simulink model "FORMATION_CONTROL_trajectory"  (R2024a)
settings: Solver=VariableStepAuto  StartTime=0.0  StopTime=100  RelTol=1e-3
undefined symbols (not defined in the file or in its folder): control_attituded_FO, control_attituded_FO2, control_attituded_FO3, control_position_FO, control_position_FO2, control_position_FO3, Decoupling, Dynamic_UAV, Dynamic_UAV1, Dynamic_UAV2
settings Model: Creator=user  LastModifiedBy=PC05
settings DebuggingCC: UnconnectedInputMsg=warning  UnconnectedOutputMsg=warning  UnconnectedLineMsg=warning
settings ModelReferenceCC: EnableRefExpFcnMdlSchedulingChecks=on
settings RTWCC: GPUComputeCapability=3.5  DLArmComputeVersion=19.05

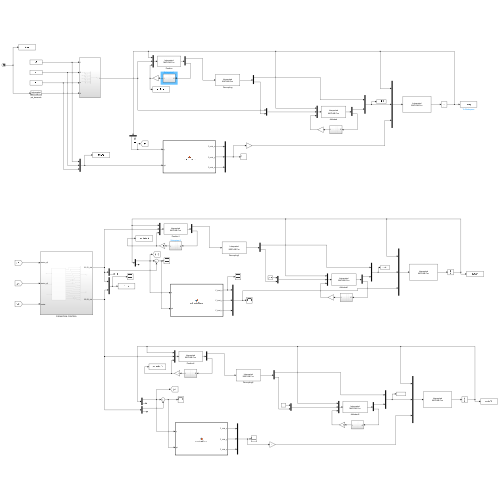
[thumbnail: Simulink's stored preview of the top-level diagram]
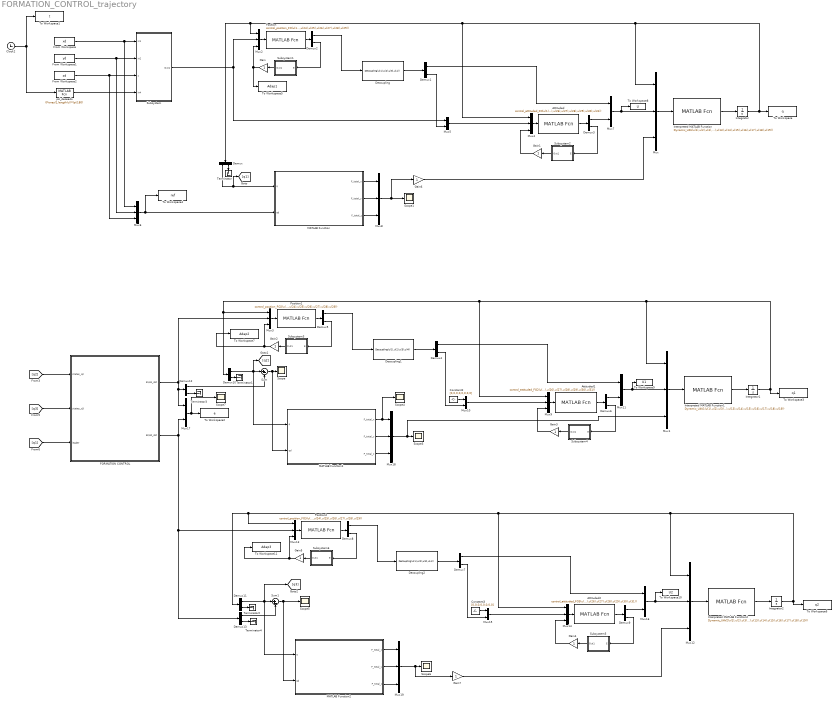
== system FORMATION_CONTROL_trajectory ==
  Attituded : MATLABFcn  MATLABFcn=control_attituded_FO(u(1),u(2),u(3),u(4),u(5),u(6),u(7),u(8),u(9),u(10),u(11),u(12),u(13),u(14),u(15),u(16),u(17),u(18),u(19),u(20),u(21),u(22),u(23),u(24),u(25),u(26),u(27),u(28),u(29),u(30),u(31))  OutputDimensions=9
  Attituded1 : MATLABFcn  MATLABFcn=control_attituded_FO2(u(1),u(2),u(3),u(4),u(5),u(6),u(7),u(8),u(9),u(10),u(11),u(12),u(13),u(14),u(15),u(16),u(17),u(18),u(19),u(20),u(21),u(22),u(23),u(24),u(25),u(26),u(27),u(28),u(29),u(30),u(31))  OutputDimensions=9
  Attituded2 : MATLABFcn  MATLABFcn=control_attituded_FO3(u(1),u(2),u(3),u(4),u(5),u(6),u(7),u(8),u(9),u(10),u(11),u(12),u(13),u(14),u(15),u(16),u(17),u(18),u(19),u(20),u(21),u(22),u(23),u(24),u(25),u(26),u(27),u(28),u(29),u(30),u(31))  OutputDimensions=9
  Clock2 : Clock
  Constant2 : Constant  Value=[0,0,0,0,0,0,0,0]
  Constant3 : Constant  Value=[0,0,0,0,0,0,0,0]
  Decoupling : MATLABFcn  MATLABFcn=Decoupling(u(1),u(2),u(3),u(4))  OutputDimensions=3
  Decoupling1 : MATLABFcn  MATLABFcn=Decoupling(u(1),u(2),u(3),u(4))  OutputDimensions=3
  Decoupling2 : MATLABFcn  MATLABFcn=Decoupling(u(1),u(2),u(3),u(4))  OutputDimensions=3
  Demux : Demux  Outputs=[6 6]
  Demux1 : Demux  Outputs=[1 2]
  Demux10 : Demux  Outputs=[6 6]
  Demux11 : Demux  Outputs=[6 6]
  Demux12 : Demux  Outputs=[6 2]
  Demux13 : Demux  Outputs=[6 2]
  Demux2 : Demux  Outputs=[4 6]
  Demux3 : Demux  Outputs=[3 6]
  Demux4 : Demux  Outputs=[1 2]
  Demux5 : Demux  Outputs=[4 6]
  Demux6 : Demux  Outputs=[3 6]
  Demux7 : Demux  Outputs=[1 2]
  Demux8 : Demux  Outputs=[4 6]
  Demux9 : Demux  Outputs=[3 6]
  FORMATION CONTROL : Subsystem
  From Workspace : FromWorkspace  VariableName=xd  OutDataTypeStr=double
  From Workspace1 : FromWorkspace  VariableName=yd  OutDataTypeStr=double
  From Workspace2 : FromWorkspace  VariableName=zd  OutDataTypeStr=double
  Gain{,1..7} (8 alike) : Gain
  Integrator : Integrator  InitialCondition=[0.5 0.5 0.01 0.01 0.01 0.01 0.01 0.01 0.05 0.01 0.01 0.01]
  Integrator1 : Integrator  InitialCondition=[-1 -2 0.01 0.01 0.01 0.01 0.01 0.01 0.05 0.01 0.01 0.01]
  Integrator2 : Integrator  InitialCondition=[-1 2 0.01 0.01 0.01 0.01 0.01 0.01 0.05 0.01 0.01 0.01]
  Interpreted MATLAB Function : MATLABFcn  MATLABFcn=Dynamic_UAV(u(1),u(2),u(3),u(4),u(5),u(6),u(7),u(8),u(9),u(10),u(11),u(12),u(13),u(14),u(15),u(16),u(17),u(18),u(19))  OutputDimensions=12
  Interpreted MATLAB Function1 : MATLABFcn  MATLABFcn=Dynamic_UAV1(u(1),u(2),u(3),u(4),u(5),u(6),u(7),u(8),u(9),u(10),u(11),u(12),u(13),u(14),u(15),u(16),u(17),u(18),u(19))  OutputDimensions=12
  Interpreted MATLAB Function2 : MATLABFcn  MATLABFcn=Dynamic_UAV2(u(1),u(2),u(3),u(4),u(5),u(6),u(7),u(8),u(9),u(10),u(11),u(12),u(13),u(14),u(15),u(16),u(17),u(18),u(19))  OutputDimensions=12
  MATLAB Function : MATLAB Function  TreatAsAtomicUnit=on
  MATLAB Function1 : MATLAB Function  TreatAsAtomicUnit=on
  MATLAB Function2 : MATLAB Function  TreatAsAtomicUnit=on
  Mux : Mux  Inputs=[12 4 3]
  Mux1 : Mux  Inputs=[12 4 3]
  Mux10 : Mux  Inputs=[8 2]
  Mux11 : Mux  Inputs=[1 3]
  Mux12 : Mux  Inputs=[12 4 3]
  Mux13 : Mux  Inputs=[12 8 9]
  Mux14 : Mux  Inputs=[12 10 9]
  Mux15 : Mux  Inputs=[8 2]
  Mux16 : Mux  Inputs=[1 3]
  Mux17 : Mux  Inputs=2
  Mux{6,8,18..19} (4 alike) : Mux  Inputs=3
  Mux2 : Mux  Inputs=[12 8 9]
  Mux3 : Mux  Inputs=[12 8 9]
  Mux4 : Mux  Inputs=[12 10 9]
  Mux5 : Mux  Inputs=[8 2]
  Mux7 : Mux  Inputs=[1 3]
  Mux9 : Mux  Inputs=[12 10 9]
  Position : MATLABFcn  MATLABFcn=control_position_FO(u(1),u(2),u(3),u(4),u(5),u(6),u(7),u(8),u(9),u(10),u(11),u(12),u(13),u(14),u(15),u(16),u(17),u(18),u(19),u(20),u(21),u(22),u(23),u(24),u(25),u(26),u(27),u(28),u(29))  OutputDimensions=10
  Position1 : MATLABFcn  MATLABFcn=control_position_FO2(u(1),u(2),u(3),u(4),u(5),u(6),u(7),u(8),u(9),u(10),u(11),u(12),u(13),u(14),u(15),u(16),u(17),u(18),u(19),u(20),u(21),u(22),u(23),u(24),u(25),u(26),u(27),u(28),u(29))  OutputDimensions=10
  Position2 : MATLABFcn  MATLABFcn=control_position_FO3(u(1),u(2),u(3),u(4),u(5),u(6),u(7),u(8),u(9),u(10),u(11),u(12),u(13),u(14),u(15),u(16),u(17),u(18),u(19),u(20),u(21),u(22),u(23),u(24),u(25),u(26),u(27),u(28),u(29))  OutputDimensions=10
  Scope{,1,3..7} (7 alike) : Scope
  Subsystem : Subsystem
  Subsystem1 : Subsystem
  Subsystem2 : Subsystem
  Subsystem3 : Subsystem
  Subsystem4 : Subsystem
  Subsystem5 : Subsystem
  Subsystem6 : Subsystem
  Sum : Sum  Inputs=|+-
  Sum1 : Sum  Inputs=|+-
  Terminator{,1..4} (5 alike) : Terminator
  To Workspace : ToWorkspace  VariableName=q  SampleTime=-1
  To Workspace1 : ToWorkspace  VariableName=t  SampleTime=-1
  To Workspace10 : ToWorkspace  VariableName=U2  SampleTime=-1
  To Workspace11 : ToWorkspace  VariableName=Adap3  SampleTime=-1
  To Workspace2 : ToWorkspace  VariableName=e  SampleTime=-1
  To Workspace3 : ToWorkspace  VariableName=q1  SampleTime=-1
  To Workspace4 : ToWorkspace  VariableName=ref  SampleTime=-1
  To Workspace5 : ToWorkspace  VariableName=Adap1  SampleTime=-1
  To Workspace6 : ToWorkspace  VariableName=q2  SampleTime=-1
  To Workspace7 : ToWorkspace  VariableName=Adap2  SampleTime=-1
  To Workspace8 : ToWorkspace  VariableName=U  SampleTime=-1
  To Workspace9 : ToWorkspace  VariableName=U1  SampleTime=-1
  psi_deseado : MATLABFcn  MATLABFcn=0*ones(1,length(u))*(pi/180)
  wires:
  Mux/1 -> Interpreted MATLAB Function/1
  Interpreted MATLAB Function/1 -> Integrator/1
  Integrator/1 -> To Workspace/1, Demux/1, Mux2/1, Mux4/1, Mux/1
  From Workspace/1 -> Subsystem/1(In1), Mux6/1
  From Workspace1/1 -> Mux6/2, Subsystem/2(In2)
  From Workspace2/1 -> Subsystem/3(z), Mux6/3
  psi_deseado/1 -> Subsystem/4(In4)
  Mux2/1 -> Position/1
  Decoupling/1 -> Demux1/1
  Mux5/1 -> Mux4/2
  Demux1/1 -> Mux7/1
  Mux7/1 -> To Workspace8/1, Mux/2
  Demux1/2 -> Mux5/2
  Clock2/1 -> psi_deseado/1, To Workspace1/1
  Demux/2 -> Terminator/1
  Demux/1 -> [q1], MATLAB Function/1(q)
  Mux6/1 -> To Workspace4/1, MATLAB Function/2(qd)
  MATLAB Function/1(F_total_x) -> Mux8/1
  MATLAB Function/2(F_total_y) -> Mux8/2
  MATLAB Function/3(F_total_z) -> Mux8/3
  Demux2/1 -> Decoupling/1
  Position/1 -> Demux2/1
  Mux4/1 -> Attituded/1
  Attituded/1 -> Demux3/1
  Demux3/1 -> Mux7/2
  [q1] -> FORMATION CONTROL/3(leader)
  [q3] -> FORMATION CONTROL/2(states_q3)
  [q2] -> FORMATION CONTROL/1(states_q2)
  Decoupling1/1 -> Demux4/1
  Interpreted MATLAB Function1/1 -> Integrator1/1
  Mux1/1 -> Interpreted MATLAB Function1/1
  Demux4/1 -> Mux11/1
  Mux18/1 -> Mux1/3, Scope3/1
  Demux4/2 -> Mux10/2
  Mux11/1 -> To Workspace9/1, Mux1/2
  Decoupling2/1 -> Demux7/1
  Interpreted MATLAB Function2/1 -> Integrator2/1
  Subsystem/1(Out1) -> Mux5/1, Mux2/2
  Mux12/1 -> Interpreted MATLAB Function2/1
  Demux7/1 -> Mux16/1
  Mux19/1 -> Gain7/1, Scope6/1
  Demux7/2 -> Mux15/2
  Mux16/1 -> Mux12/2, To Workspace10/1
  Demux10/2 -> Terminator1/1
  Demux10/1 -> MATLAB Function1/1(q), [q2], Sum/1
  Demux11/1 -> MATLAB Function2/1(q), [q3], Sum1/1
  Demux11/2 -> Terminator2/1
  Constant2/1 -> Mux10/1
  Constant3/1 -> Mux15/1
  Mux17/1 -> Scope7/1, To Workspace2/1
  Sum/1 -> MATLAB Function1/2(qd), Scope/1
  Demux12/1 -> Sum/2
  Demux12/2 -> Terminator3/1
  MATLAB Function1/2(F_total_y) -> Mux18/2
  MATLAB Function1/1(F_total_x) -> Scope4/1, Mux18/1
  MATLAB Function1/3(F_total_z) -> Mux18/3
  Demux13/2 -> Terminator4/1
  Sum1/1 -> MATLAB Function2/2(qd), Scope5/1
  Demux13/1 -> Sum1/2
  MATLAB Function2/2(F_total_y) -> Mux19/2
  MATLAB Function2/3(F_total_z) -> Mux19/3
  MATLAB Function2/1(F_total_x) -> Mux19/1
  Demux2/2 -> Subsystem1/1(E)
  Subsystem1/1(Out1) -> Gain/1
  Gain/1 -> To Workspace5/1, Mux2/3
  Subsystem2/1(Out1) -> Gain1/1
  Demux3/2 -> Subsystem2/1(E)
  Gain1/1 -> Mux4/3
  Subsystem3/1(Out1) -> Gain2/1
  Gain2/1 -> To Workspace7/1, Mux3/3
  FORMATION CONTROL/1(E1,E1_dot) -> Demux12/1, Mux17/1, Mux3/2
  Position1/1 -> Demux5/1
  Mux3/1 -> Position1/1
  Demux5/2 -> Subsystem3/1(E)
  Demux5/1 -> Decoupling1/1
  Gain3/1 -> Mux9/3
  Demux6/1 -> Mux11/2
  Demux6/2 -> Subsystem4/1(E)
  Mux9/1 -> Attituded1/1
  Attituded1/1 -> Demux6/1
  Subsystem4/1(Out1) -> Gain3/1
  Mux10/1 -> Mux9/2
  Integrator1/1 -> To Workspace3/1, Mux9/1, Mux3/1, Demux10/1, Mux1/1
  Gain4/1 -> Mux14/3
  Demux9/1 -> Mux16/2
  Demux9/2 -> Subsystem5/1(E)
  Mux14/1 -> Attituded2/1
  Attituded2/1 -> Demux9/1
  Subsystem5/1(Out1) -> Gain4/1
  Mux15/1 -> Mux14/2
  FORMATION CONTROL/2(E2,E2_dot) -> Demux13/1, Mux13/2, Mux17/2
  Integrator2/1 -> To Workspace6/1, Mux14/1, Mux13/1, Demux11/1, Mux12/1
  Mux13/1 -> Position2/1
  Demux8/2 -> Subsystem6/1(E)
  Demux8/1 -> Decoupling2/1
  Gain5/1 -> To Workspace11/1, Mux13/3
  Position2/1 -> Demux8/1
  Subsystem6/1(Out1) -> Gain5/1
  Mux8/1 -> Scope1/1, Gain6/1
  Gain6/1 -> Mux/3
  Gain7/1 -> Mux12/3

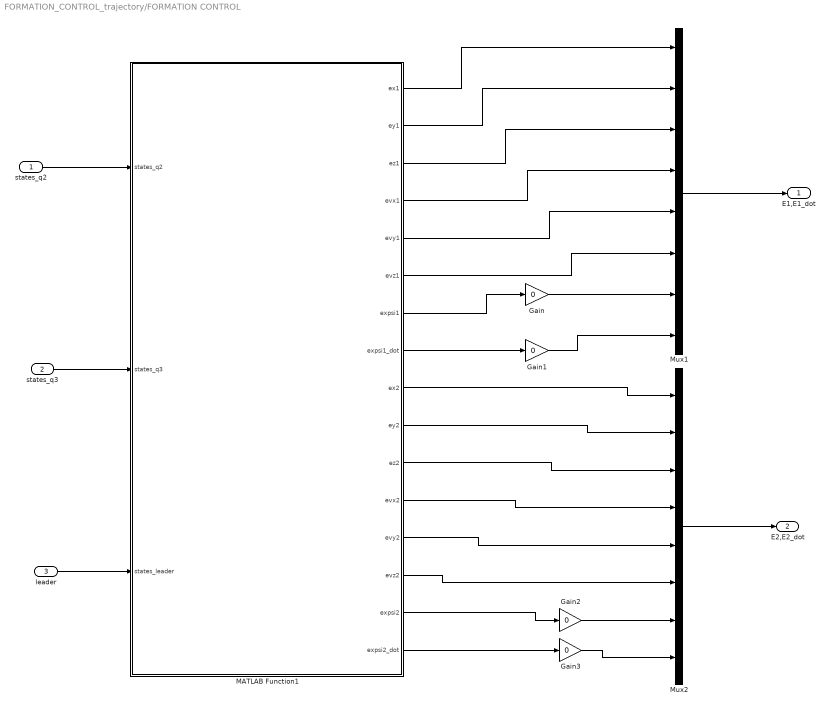
== system FORMATION_CONTROL_trajectory/FORMATION CONTROL ==
  states_q2 : Inport
  states_q3 : Inport  Port=2
  leader : Inport  Port=3
  Gain{,1..3} (4 alike) : Gain  Gain=0
  MATLAB Function1 : MATLAB Function  TreatAsAtomicUnit=on
  Mux1 : Mux  Inputs=8
  Mux2 : Mux  Inputs=8
  E1,E1_dot : Outport
  E2,E2_dot : Outport  Port=2
  wires:
  Mux1/1 -> E1,E1_dot/1
  states_q2/1 -> MATLAB Function1/1(states_q2)
  states_q3/1 -> MATLAB Function1/2(states_q3)
  leader/1 -> MATLAB Function1/3(states_leader)
  MATLAB Function1/1(ex1) -> Mux1/1
  MATLAB Function1/2(ey1) -> Mux1/2
  MATLAB Function1/3(ez1) -> Mux1/3
  MATLAB Function1/4(evx1) -> Mux1/4
  MATLAB Function1/5(evy1) -> Mux1/5
  MATLAB Function1/6(evz1) -> Mux1/6
  MATLAB Function1/14(evz2) -> Mux2/6
  MATLAB Function1/11(ez2) -> Mux2/3
  MATLAB Function1/9(ex2) -> Mux2/1
  MATLAB Function1/12(evx2) -> Mux2/4
  Mux2/1 -> E2,E2_dot/1
  MATLAB Function1/10(ey2) -> Mux2/2
  MATLAB Function1/13(evy2) -> Mux2/5
  MATLAB Function1/7(expsi1) -> Gain/1
  MATLAB Function1/8(expsi1_dot) -> Gain1/1
  MATLAB Function1/15(expsi2) -> Gain2/1
  MATLAB Function1/16(expsi2_dot) -> Gain3/1
  Gain/1 -> Mux1/7
  Gain1/1 -> Mux1/8
  Gain2/1 -> Mux2/7
  Gain3/1 -> Mux2/8

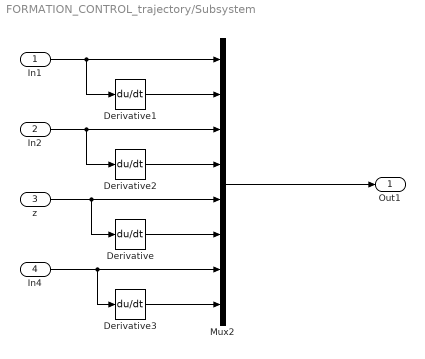
== system FORMATION_CONTROL_trajectory/Subsystem ==
  In1 : Inport
  In2 : Inport  Port=2
  z : Inport  Port=3
  In4 : Inport  Port=4
  Derivative{,1..3} (4 alike) : Derivative
  Mux2 : Mux  Inputs=8
  Out1 : Outport
  wires:
  In2/1 -> Mux2/3, Derivative2/1
  Derivative/1 -> Mux2/6
  z/1 -> Mux2/5, Derivative/1
  Derivative3/1 -> Mux2/8
  In4/1 -> Mux2/7, Derivative3/1
  In1/1 -> Mux2/1, Derivative1/1
  Derivative2/1 -> Mux2/4
  Derivative1/1 -> Mux2/2
  Mux2/1 -> Out1/1

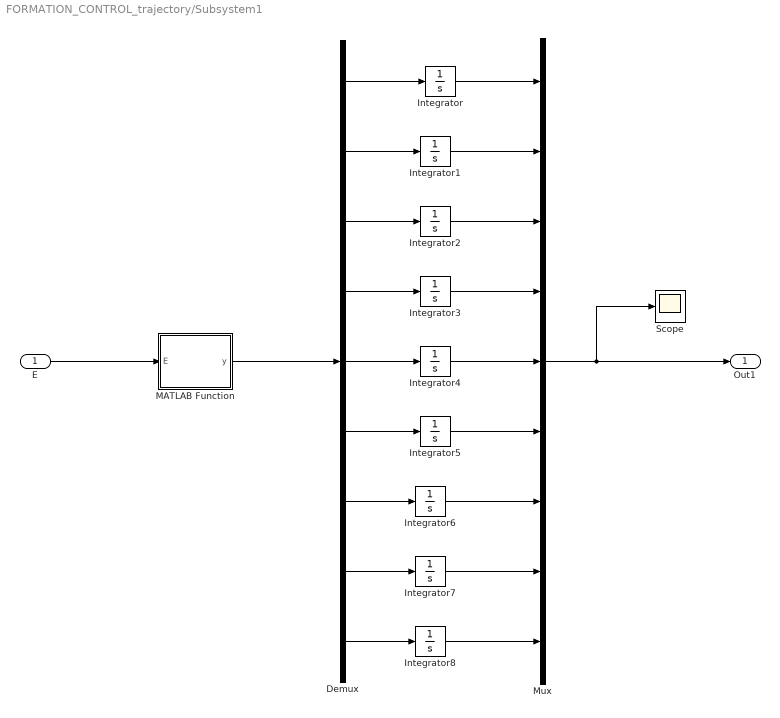
== system FORMATION_CONTROL_trajectory/Subsystem1 ==
  E : Inport
  Demux : Demux  Outputs=9
  Integrator{,1..8} (9 alike) : Integrator  InitialCondition=0.01
  MATLAB Function : MATLAB Function  TreatAsAtomicUnit=on
  Mux : Mux  Inputs=9
  Scope : Scope
  Out1 : Outport
  wires:
  Mux/1 -> Scope/1, Out1/1
  E/1 -> MATLAB Function/1(E)
  MATLAB Function/1(y) -> Demux/1
  Integrator/1 -> Mux/1
  Demux/1 -> Integrator/1
  Demux/2 -> Integrator1/1
  Integrator1/1 -> Mux/2
  Demux/3 -> Integrator2/1
  Integrator2/1 -> Mux/3
  Demux/4 -> Integrator3/1
  Integrator3/1 -> Mux/4
  Demux/5 -> Integrator4/1
  Integrator4/1 -> Mux/5
  Demux/6 -> Integrator5/1
  Integrator5/1 -> Mux/6
  Demux/7 -> Integrator6/1
  Integrator6/1 -> Mux/7
  Demux/8 -> Integrator7/1
  Integrator7/1 -> Mux/8
  Demux/9 -> Integrator8/1
  Integrator8/1 -> Mux/9

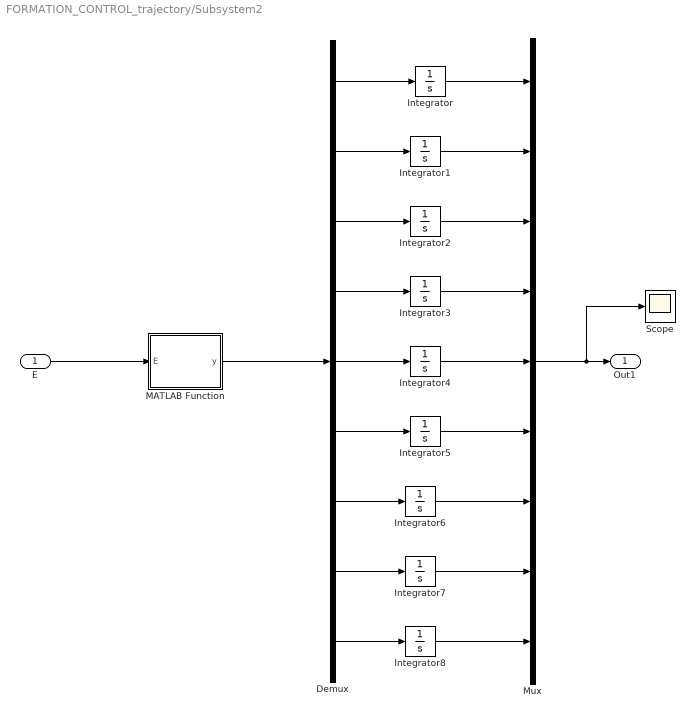
== system FORMATION_CONTROL_trajectory/Subsystem2 ==
  E : Inport
  Demux : Demux  Outputs=9
  Integrator{,1..8} (9 alike) : Integrator  InitialCondition=0.01
  MATLAB Function : MATLAB Function  TreatAsAtomicUnit=on
  Mux : Mux  Inputs=9
  Scope : Scope
  Out1 : Outport
  wires:
  Demux/5 -> Integrator4/1
  Integrator3/1 -> Mux/4
  Integrator6/1 -> Mux/7
  Demux/8 -> Integrator7/1
  Integrator5/1 -> Mux/6
  Integrator4/1 -> Mux/5
  Demux/9 -> Integrator8/1
  Demux/6 -> Integrator5/1
  Integrator8/1 -> Mux/9
  Integrator7/1 -> Mux/8
  Demux/7 -> Integrator6/1
  Demux/4 -> Integrator3/1
  Integrator2/1 -> Mux/3
  Demux/3 -> Integrator2/1
  Demux/1 -> Integrator/1
  Mux/1 -> Scope/1, Out1/1
  Integrator/1 -> Mux/1
  Integrator1/1 -> Mux/2
  Demux/2 -> Integrator1/1
  E/1 -> MATLAB Function/1(E)
  MATLAB Function/1(y) -> Demux/1

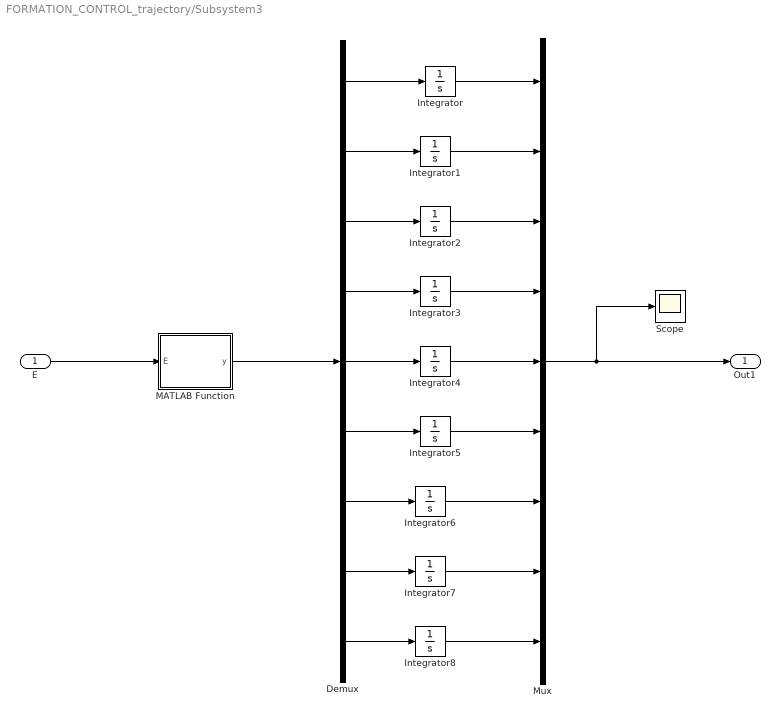
== system FORMATION_CONTROL_trajectory/Subsystem3 ==
  E : Inport
  Demux : Demux  Outputs=9
  Integrator{,1..8} (9 alike) : Integrator  InitialCondition=0.01
  MATLAB Function : MATLAB Function  TreatAsAtomicUnit=on
  Mux : Mux  Inputs=9
  Scope : Scope
  Out1 : Outport
  wires:
  Mux/1 -> Scope/1, Out1/1
  E/1 -> MATLAB Function/1(E)
  MATLAB Function/1(y) -> Demux/1
  Integrator/1 -> Mux/1
  Demux/1 -> Integrator/1
  Demux/2 -> Integrator1/1
  Integrator1/1 -> Mux/2
  Demux/3 -> Integrator2/1
  Integrator2/1 -> Mux/3
  Demux/4 -> Integrator3/1
  Integrator3/1 -> Mux/4
  Demux/5 -> Integrator4/1
  Integrator4/1 -> Mux/5
  Demux/6 -> Integrator5/1
  Integrator5/1 -> Mux/6
  Demux/7 -> Integrator6/1
  Integrator6/1 -> Mux/7
  Demux/8 -> Integrator7/1
  Integrator7/1 -> Mux/8
  Demux/9 -> Integrator8/1
  Integrator8/1 -> Mux/9

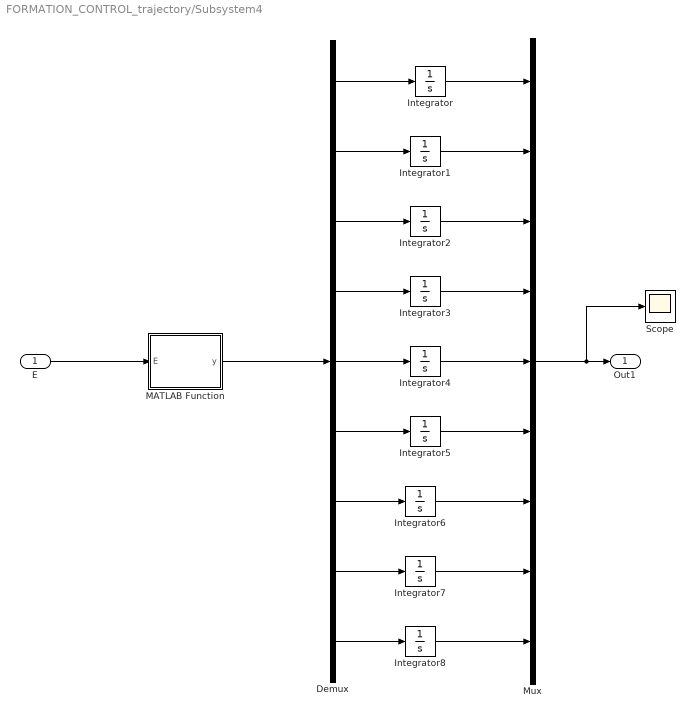
== system FORMATION_CONTROL_trajectory/Subsystem4 ==
  E : Inport
  Demux : Demux  Outputs=9
  Integrator{,1..8} (9 alike) : Integrator  InitialCondition=0.01
  MATLAB Function : MATLAB Function  TreatAsAtomicUnit=on
  Mux : Mux  Inputs=9
  Scope : Scope
  Out1 : Outport
  wires:
  Demux/5 -> Integrator4/1
  Integrator3/1 -> Mux/4
  Integrator6/1 -> Mux/7
  Demux/8 -> Integrator7/1
  Integrator5/1 -> Mux/6
  Integrator4/1 -> Mux/5
  Demux/9 -> Integrator8/1
  Demux/6 -> Integrator5/1
  Integrator8/1 -> Mux/9
  Integrator7/1 -> Mux/8
  Demux/7 -> Integrator6/1
  Demux/4 -> Integrator3/1
  Integrator2/1 -> Mux/3
  Demux/3 -> Integrator2/1
  Demux/1 -> Integrator/1
  Mux/1 -> Scope/1, Out1/1
  Integrator/1 -> Mux/1
  Integrator1/1 -> Mux/2
  Demux/2 -> Integrator1/1
  E/1 -> MATLAB Function/1(E)
  MATLAB Function/1(y) -> Demux/1

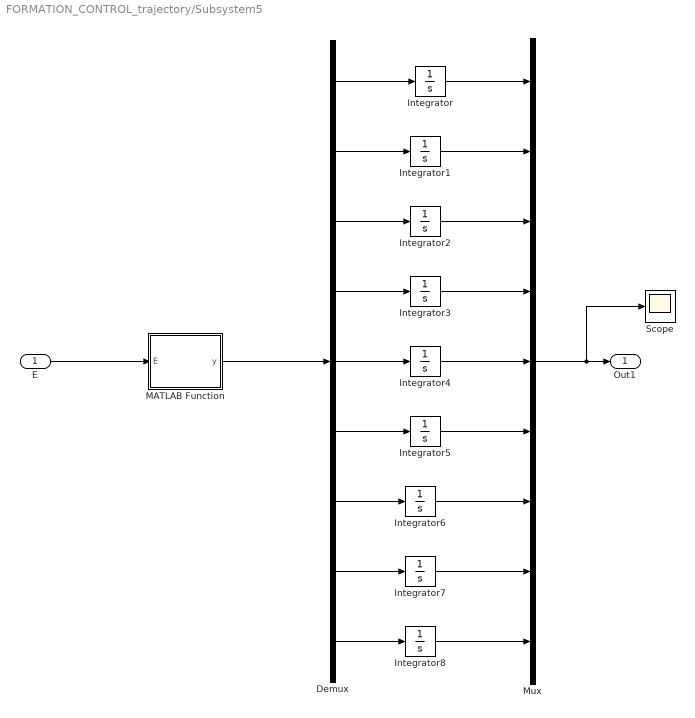
== system FORMATION_CONTROL_trajectory/Subsystem5 ==
  E : Inport
  Demux : Demux  Outputs=9
  Integrator{,1..8} (9 alike) : Integrator  InitialCondition=0.01
  MATLAB Function : MATLAB Function  TreatAsAtomicUnit=on
  Mux : Mux  Inputs=9
  Scope : Scope
  Out1 : Outport
  wires:
  Demux/5 -> Integrator4/1
  Integrator3/1 -> Mux/4
  Integrator6/1 -> Mux/7
  Demux/8 -> Integrator7/1
  Integrator5/1 -> Mux/6
  Integrator4/1 -> Mux/5
  Demux/9 -> Integrator8/1
  Demux/6 -> Integrator5/1
  Integrator8/1 -> Mux/9
  Integrator7/1 -> Mux/8
  Demux/7 -> Integrator6/1
  Demux/4 -> Integrator3/1
  Integrator2/1 -> Mux/3
  Demux/3 -> Integrator2/1
  Demux/1 -> Integrator/1
  Mux/1 -> Scope/1, Out1/1
  Integrator/1 -> Mux/1
  Integrator1/1 -> Mux/2
  Demux/2 -> Integrator1/1
  E/1 -> MATLAB Function/1(E)
  MATLAB Function/1(y) -> Demux/1

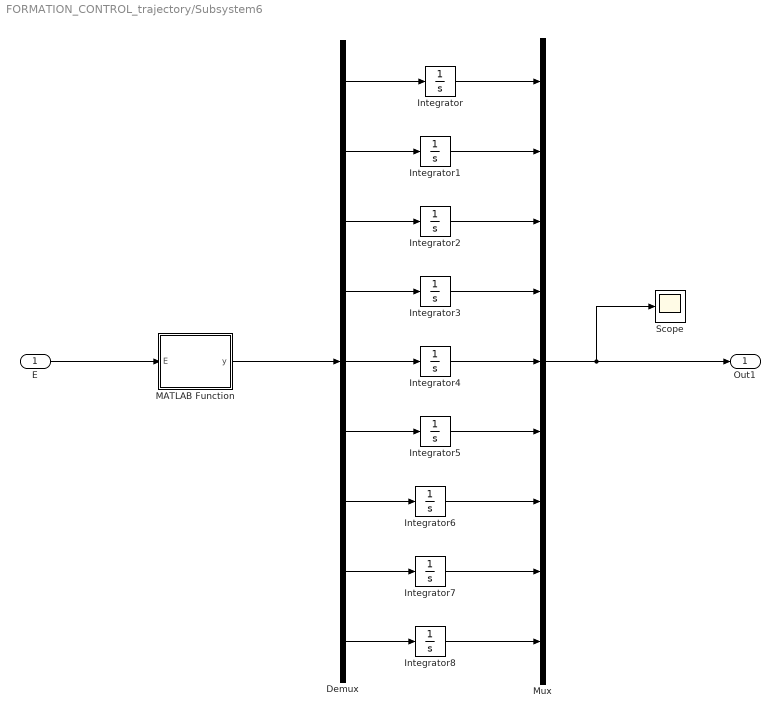
== system FORMATION_CONTROL_trajectory/Subsystem6 ==
  E : Inport
  Demux : Demux  Outputs=9
  Integrator{,1..8} (9 alike) : Integrator  InitialCondition=0.01
  MATLAB Function : MATLAB Function  TreatAsAtomicUnit=on
  Mux : Mux  Inputs=9
  Scope : Scope
  Out1 : Outport
  wires:
  Mux/1 -> Scope/1, Out1/1
  E/1 -> MATLAB Function/1(E)
  MATLAB Function/1(y) -> Demux/1
  Integrator/1 -> Mux/1
  Demux/1 -> Integrator/1
  Demux/2 -> Integrator1/1
  Integrator1/1 -> Mux/2
  Demux/3 -> Integrator2/1
  Integrator2/1 -> Mux/3
  Demux/4 -> Integrator3/1
  Integrator3/1 -> Mux/4
  Demux/5 -> Integrator4/1
  Integrator4/1 -> Mux/5
  Demux/6 -> Integrator5/1
  Integrator5/1 -> Mux/6
  Demux/7 -> Integrator6/1
  Integrator6/1 -> Mux/7
  Demux/8 -> Integrator7/1
  Integrator7/1 -> Mux/8
  Demux/9 -> Integrator8/1
  Integrator8/1 -> Mux/9

== matlab function FORMATION_CONTROL_trajectory/MATLAB Function2 ==
  data: q input; F_total_x output; qd input; F_total_y output; F_total_z output
function [F_total_x, F_total_y, F_total_z] = calculateFtotal(q, qd)
    % q: Posición actual del cuadricóptero [x, y, z]
    % qd: Posición de referencia [xd, yd, zd]
    % obs: Posición de los obstáculos [xo, yo, zo]
    % k_att: Constante de proporcionalidad para la fuerza atractiva
    % k_rep: Constante de proporcionalidad para la fuerza repulsiva
    % rho_0: Umbral de influencia del obstáculo
    
    k_att = 3; % constante del campo atractivo
    k_repx = 0.5; % constante del campo repulsivo
    k_repy = 0.5; % constante del campo repulsivo
    k_repz = 0; % constante del campo repulsivo
    rho_0 = 1; % radio de influencia del obstáculo

    % Definición de obstáculos (tres obstáculos)
    obstacles = [
       5.8, 3.5, 4;  % Obstacle 1
        0, 0, 0;  % Obstacle 2
        6, 13, 4   % Obstacle 3
    ];

    x = q(1);
    y = q(2);
    z = q(3);
    xd = qd(1);
    yd = qd(2);
    zd = qd(3);

    % Calcular la fuerza atractiva
    F_attX = -k_att * (x - xd);
    F_attY = -k_att * (y - yd);
    F_attZ = -k_att * (z - zd);

    % Inicializar la fuerza repulsiva a cero
    F_repX = 0;
    F_repY = 0;
    F_repZ = 0;

    % Calcular la fuerza repulsiva para cada obstáculo
    for i = 1:size(obstacles, 1)
        obs = obstacles(i, :);
        rho = sqrt((x - obs(1))^2 + (y - obs(2))^2 + (z - obs(3))^2);
        
        if rho <= rho_0
            directionX = (x - obs(1)) / rho;
            directionY = (y - obs(2)) / rho;
            directionZ = (z - obs(3)) / rho;
            F_repX = F_repX + k_repx * (1/rho - 1/rho_0) * (1/rho^2) * directionX;
            F_repY = F_repY + k_repy * (1/rho - 1/rho_0) * (1/rho^2) * directionY;
            F_repZ = F_repZ + k_repz * (1/rho - 1/rho_0) * (1/rho^2) * directionZ;
        end
    end

    F_total_x = (F_attX + F_repX);
    F_total_y = (F_attY + F_repY);
    F_total_z = (F_attZ + F_repZ);
    
end

== matlab function FORMATION_CONTROL_trajectory/FORMATION CONTROL/MATLAB Function1 ==
  data: states_q2 input; states_q3 input; states_leader input; ex1 output; ey1 output; ez1 output; evx1 output; evy1 output; evz1 output; expsi1 output; expsi1_dot output; ex2 output; ey2 output; ez2 output; evx2 output; evy2 output; evz2 output; expsi2 output; expsi2_dot output
function [ex1,ey1,ez1,evx1,evy1,evz1,expsi1,expsi1_dot,ex2,ey2,ez2,evx2,evy2,evz2,expsi2,expsi2_dot] = formation_control(states_q2,states_q3,states_leader)
x2=states_q2(1);
y2=states_q2(2);
z2=states_q2(3);
Vx2=states_q2(4);
Vy2=states_q2(5);
Vz2=states_q2(6);
x3=states_q3(1);
y3=states_q3(2);
z3=states_q3(3);
Vx3=states_q3(4);
Vy3=states_q3(5);
Vz3=states_q3(6);
x0=states_leader(1);
y0=states_leader(2);
z0=states_leader(3);
Vx0=states_leader(4);
Vy0=states_leader(5);
Vz0=states_leader(6);


p=[x2,y2,z2,x3,y3,z3]';
v=[Vx2,Vy2,Vz2,Vx3,Vy3,Vz3]';
p0=[x0 y0 z0]';
v0=[Vx0 Vy0 Vz0]';
h1=[0, -1, 0];
h2=[ 0, 1, 0];
h=[h1,h2]';
L=[0 0;-1 1];
B=[1 0; 0 0];
LB=L+B;
p_=p - kron(ones(2,1),p0) - h;
ep_=p_;

v_= v - kron(ones(2,1),v0);
ev_=v_;

ex1=ep_(1);
ey1=ep_(2);
ez1=ep_(3);
evx1=ev_(1);
evy1=ev_(2);
evz1=ev_(3);
expsi1=ex1*0;
expsi1_dot=ex1*0;


ex2=ep_(4);
ey2=ep_(5);
ez2=ep_(6);
evx2=ev_(4);
evy2=ev_(5);
evz2=ev_(6);
expsi2=ex2*0;
expsi2_dot=ex2*0;
end

== matlab function FORMATION_CONTROL_trajectory/MATLAB Function1 ==
  data: q input; F_total_x output; qd input; F_total_y output; F_total_z output
function [F_total_x, F_total_y, F_total_z] = calculateFtotal(q, qd)
    % q: Posición actual del cuadricóptero [x, y, z]
    % qd: Posición de referencia [xd, yd, zd]
    % obs: Posición de los obstáculos [xo, yo, zo]
    % k_att: Constante de proporcionalidad para la fuerza atractiva
    % k_rep: Constante de proporcionalidad para la fuerza repulsiva
    % rho_0: Umbral de influencia del obstáculo
    
    k_att = 3; % constante del campo atractivo
    k_repx = 0.5; % constante del campo repulsivo
    k_repy = 0.5; % constante del campo repulsivo
    k_repz = 0; % constante del campo repulsivo
    rho_0 = 1; % radio de influencia del obstáculo

    % Definición de obstáculos (tres obstáculos)
    obstacles = [
        0, 0, 0;  % Obstacle 1
        6, 8, 4;  % Obstacle 2
        0, 0, 0   % Obstacle 3
    ];

    x = q(1);
    y = q(2);
    z = q(3);
    xd = qd(1);
    yd = qd(2);
    zd = qd(3);

    % Calcular la fuerza atractiva
    F_attX = -k_att * (x - xd);
    F_attY = -k_att * (y - yd);
    F_attZ = -k_att * (z - zd);

    % Inicializar la fuerza repulsiva a cero
    F_repX = 0;
    F_repY = 0;
    F_repZ = 0;

    % Calcular la fuerza repulsiva para cada obstáculo
    for i = 1:size(obstacles, 1)
        obs = obstacles(i, :);
        rho = sqrt((x - obs(1))^2 + (y - obs(2))^2 + (z - obs(3))^2);
        
        if rho <= rho_0
            directionX = (x - obs(1)) / rho;
            directionY = (y - obs(2)) / rho;
            directionZ = (z - obs(3)) / rho;
            F_repX = F_repX + k_repx * (1/rho - 1/rho_0) * (1/rho^2) * directionX;
            F_repY = F_repY + k_repy * (1/rho - 1/rho_0) * (1/rho^2) * directionY;
            F_repZ = F_repZ + k_repz * (1/rho - 1/rho_0) * (1/rho^2) * directionZ;
        end
    end

    F_total_x = (F_attX + F_repX);
    F_total_y = (F_attY + F_repY);
    F_total_z = (F_attZ + F_repZ);
    
end

== matlab function FORMATION_CONTROL_trajectory/MATLAB Function ==
  data: q input; F_total_x output; qd input; F_total_y output; F_total_z output
function [F_total_x, F_total_y, F_total_z] = calculateFtotal(q, qd)
    % q: Posición actual del cuadricóptero [x, y, z]
    % qd: Posición de referencia [xd, yd, zd]
    % obs: Posición de los obstáculos [xo, yo, zo]
    % k_att: Constante de proporcionalidad para la fuerza atractiva
    % k_rep: Constante de proporcionalidad para la fuerza repulsiva
    % rho_0: Umbral de influencia del obstáculo
    
    k_att = 3; % constante del campo atractivo
    k_repx = 0.05; % constante del campo repulsivo
    k_repy = 0.05; % constante del campo repulsivo
    k_repz = 0; % constante del campo repulsivo
    rho_0 = 1; % radio de influencia del obstáculo

    % Definición de obstáculos (tres obstáculos)
    obstacles = [
        6, 3, 4;  % Obstacle 1
        0, 0, 0;  % Obstacle 2
        0, 0, 0   % Obstacle 3
    ];

    x = q(1);
    y = q(2);
    z = q(3);
    xd = qd(1);
    yd = qd(2);
    zd = qd(3);

    % Calcular la fuerza atractiva
    F_attX = -k_att * (x - xd);
    F_attY = -k_att * (y - yd);
    F_attZ = -k_att * (z - zd);

    % Inicializar la fuerza repulsiva a cero
    F_repX = 0;
    F_repY = 0;
    F_repZ = 0;

    % Calcular la fuerza repulsiva para cada obstáculo
    for i = 1:size(obstacles, 1)
        obs = obstacles(i, :);
        rho = sqrt((x - obs(1))^2 + (y - obs(2))^2 + (z - obs(3))^2);
        
        if rho <= rho_0
            directionX = (x - obs(1)) / rho;
            directionY = (y - obs(2)) / rho;
            directionZ = (z - obs(3)) / rho;
            F_repX = F_repX + k_repx * (1/rho - 1/rho_0) * (1/rho^2) * directionX;
            F_repY = F_repY + k_repy * (1/rho - 1/rho_0) * (1/rho^2) * directionY;
            F_repZ = F_repZ + k_repz * (1/rho - 1/rho_0) * (1/rho^2) * directionZ;
        end
    end

    F_total_x = (F_attX + F_repX);
    F_total_y = (F_attY + F_repY);
    F_total_z = (F_attZ + F_repZ);
    
end

== matlab function FORMATION_CONTROL_trajectory/Subsystem1/MATLAB Function ==
  data: E input; y output
function y = FOSMC(E)

ex=E(1);
ey=E(2);
ez=E(3);
sx=E(4);
sy=E(5);
sz=E(6);

Ix_fo=(0.05*(abs(ex)^0.3)*tanh(ex));
Iy_fo=(0.05*(abs(ey)^0.3)*tanh(ey));
Iz_fo=(0.05*(abs(ez)^0.3)*tanh(ez));
k1x_est=3*abs(sx)^(2);
k2x_est=3*abs(sx)^(1.2);
k1y_est=3*abs(sy)^(2);
k2y_est=3*abs(sy)^(1.2);
k1z_est=3*abs(sz)^(2);
k2z_est=3*abs(sz)^(1.2);

y = [Ix_fo,Iy_fo,Iz_fo,k1x_est*0.1,k2x_est*0.1,k1y_est*0.1,k2y_est*0.1,k1z_est*0.05,k2z_est*0.05];

== matlab function FORMATION_CONTROL_trajectory/Subsystem2/MATLAB Function ==
  data: E input; y output
function y = FOSMC(E)

ex=E(1);
ey=E(2);
ez=E(3);
sx=E(4);
sy=E(5);
sz=E(6);

Ix_fo=(0.0002*(abs(ex)^1.2)*tanh(ex));
Iy_fo=(0.0002*(abs(ey)^1.2)*tanh(ey));
Iz_fo=(0.0002*(abs(ez)^1.2)*tanh(ez));
k1x_est=2*abs(sx)^(2);
k2x_est=1.67*abs(sx)^(1.2);
k1y_est=2*abs(sy)^(2);
k2y_est=1.67*abs(sy)^(1.2);
k1z_est=2*abs(sz)^(2);
k2z_est=1.67*abs(sz)^(1.2);

y = [Ix_fo,Iy_fo,Iz_fo,1*k1x_est,1*k2x_est,1*k1y_est,1*k2y_est,1*k1z_est,1*k2z_est];

== matlab function FORMATION_CONTROL_trajectory/Subsystem3/MATLAB Function ==
  data: E input; y output
function y = FOSMC(E)

ex=E(1);
ey=E(2);
ez=E(3);
sx=E(4);
sy=E(5);
sz=E(6);

Ix_fo=(0.05*(abs(ex)^0.3)*tanh(ex));
Iy_fo=(0.05*(abs(ey)^0.3)*tanh(ey));
Iz_fo=(0.05*(abs(ez)^0.3)*tanh(ez));
k1x_est=3*abs(sx)^(2);
k2x_est=3*abs(sx)^(1.2);
k1y_est=3*abs(sy)^(2);
k2y_est=3*abs(sy)^(1.2);
k1z_est=3*abs(sz)^(2);
k2z_est=3*abs(sz)^(1.2);

y = [Ix_fo,Iy_fo,Iz_fo,k1x_est*0.1,k2x_est*0.1,k1y_est*0.1,k2y_est*0.1,k1z_est*0.05,k2z_est*0.05];

== matlab function FORMATION_CONTROL_trajectory/Subsystem4/MATLAB Function ==
  data: E input; y output
function y = FOSMC(E)

ex=E(1);
ey=E(2);
ez=E(3);
sx=E(4);
sy=E(5);
sz=E(6);

Ix_fo=(0.0002*(abs(ex)^1.2)*tanh(ex));
Iy_fo=(0.0002*(abs(ey)^1.2)*tanh(ey));
Iz_fo=(0.0002*(abs(ez)^1.2)*tanh(ez));
k1x_est=2*abs(sx)^(2);
k2x_est=1.67*abs(sx)^(1.2);
k1y_est=2*abs(sy)^(2);
k2y_est=1.67*abs(sy)^(1.2);
k1z_est=2*abs(sz)^(2);
k2z_est=1.67*abs(sz)^(1.2);

y = [Ix_fo,Iy_fo,Iz_fo,1*k1x_est,1*k2x_est,1*k1y_est,1*k2y_est,1*k1z_est,1*k2z_est];

== matlab function FORMATION_CONTROL_trajectory/Subsystem5/MATLAB Function ==
  data: E input; y output
function y = FOSMC(E)

ex=E(1);
ey=E(2);
ez=E(3);
sx=E(4);
sy=E(5);
sz=E(6);

Ix_fo=(0.0002*(abs(ex)^1.2)*tanh(ex));
Iy_fo=(0.0002*(abs(ey)^1.2)*tanh(ey));
Iz_fo=(0.0002*(abs(ez)^1.2)*tanh(ez));
k1x_est=2*abs(sx)^(2);
k2x_est=1.67*abs(sx)^(1.2);
k1y_est=2*abs(sy)^(2);
k2y_est=1.67*abs(sy)^(1.2);
k1z_est=2*abs(sz)^(2);
k2z_est=1.67*abs(sz)^(1.2);

y = [Ix_fo,Iy_fo,Iz_fo,1*k1x_est,1*k2x_est,1*k1y_est,1*k2y_est,1*k1z_est,1*k2z_est];

== matlab function FORMATION_CONTROL_trajectory/Subsystem6/MATLAB Function ==
  data: E input; y output
function y = FOSMC(E)

ex=E(1);
ey=E(2);
ez=E(3);
sx=E(4);
sy=E(5);
sz=E(6);

Ix_fo=(0.05*(abs(ex)^0.3)*tanh(ex));
Iy_fo=(0.05*(abs(ey)^0.3)*tanh(ey));
Iz_fo=(0.05*(abs(ez)^0.3)*tanh(ez));
k1x_est=3*abs(sx)^(2);
k2x_est=3*abs(sx)^(1.2);
k1y_est=3*abs(sy)^(2);
k2y_est=3*abs(sy)^(1.2);
k1z_est=3*abs(sz)^(2);
k2z_est=3*abs(sz)^(1.2);

y = [Ix_fo,Iy_fo,Iz_fo,k1x_est*0.1,k2x_est*0.1,k1y_est*0.1,k2y_est*0.1,k1z_est*0.05,k2z_est*0.05];
